simulink model "Sistema"  (R2023a)
settings: Solver=VariableStepAuto  StartTime=0.0  StopTime=15  MaxStep=1E-3  RelTol=1e-3
libraries: fl_lib x21, nesl_utility x9, slpidlib x2
settings Model: LastModifiedBy=vania
settings DataIOCC: SaveFormat=Array  ReturnWorkspaceOutputs=off  TimeSaveName=t
settings DebuggingCC: AlgebraicLoopMsg=none  ArtificialAlgebraicLoopMsg=none  MaxConsecutiveZCsMsg=none  ModelReferenceExtraNoncontSigs=none  OperatingPointInterfaceChecksumMismatchMsg=none
settings RTWCC: GPUComputeCapability=5.0

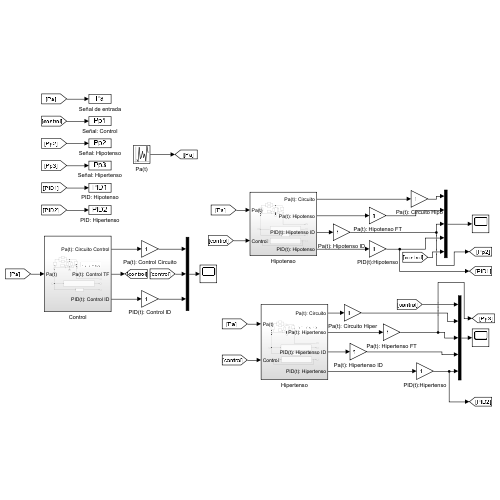
[thumbnail: Simulink's stored preview of the top-level diagram]
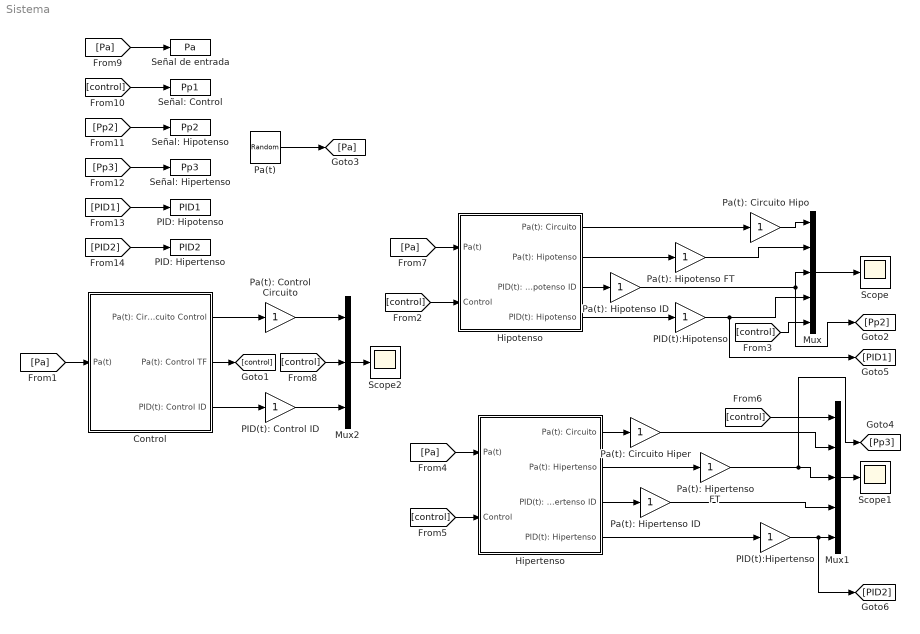
== system Sistema ==
  Control : Subsystem
  Hipertenso : Subsystem
  Hipotenso : Subsystem
  Mux : Mux  Inputs=5
  Mux1 : Mux  Inputs=5
  Mux2 : Mux  Inputs=3
  PID(t): Control ID : Gain
  PID(t):Hipertenso : Gain
  PID(t):Hipotenso : Gain
  PID: Hipertenso : ToWorkspace  VariableName=PID2  SampleTime=-1
  PID: Hipotenso : ToWorkspace  VariableName=PID1  SampleTime=-1
  Pa(t) : UniformRandomNumber  Minimum=-0.2  Seed=106  SampleTime=0.5
  Pa(t): Circuito Hiper : Gain
  Pa(t): Circuito Hipo : Gain
  Pa(t): Control Circuito : Gain
  Pa(t): Hipertenso FT : Gain
  Pa(t): Hipertenso ID : Gain
  Pa(t): Hipotenso FT : Gain
  Pa(t): Hipotenso ID : Gain
  Scope : Scope
  Scope1 : Scope
  Scope2 : Scope
  Señal de entrada : ToWorkspace  VariableName=Pa  SampleTime=-1
  Señal: Control : ToWorkspace  VariableName=Pp1  SampleTime=-1
  Señal: Hipertenso : ToWorkspace  VariableName=Pp3  SampleTime=-1
  Señal: Hipotenso : ToWorkspace  VariableName=Pp2  SampleTime=-1
  wires:
  Pa(t)/1 -> [Pa]
  Mux/1 -> Scope/1
  Hipotenso/1(Pa(t): Circuito) -> Pa(t): Circuito Hipo/1
  Hipotenso/2(Pa(t): Hipotenso) -> Pa(t): Hipotenso FT/1
  Hipotenso/3(PID(t): Hipotenso ID) -> Pa(t): Hipotenso ID/1
  Hipotenso/4(PID(t): Hipotenso) -> PID(t):Hipotenso/1
  [control] -> Hipotenso/2(Control)
  [control] -> Mux/5
  Pa(t): Hipotenso FT/1 -> Mux/2
  Pa(t): Circuito Hipo/1 -> Mux/1
  Pa(t): Hipotenso ID/1 -> Mux/3, [Pp2]
  PID(t):Hipotenso/1 -> Mux/4, [PID1]
  [Pa] -> Hipertenso/1(Pa(t))
  [control] -> Hipertenso/2(Control)
  Pa(t): Circuito Hiper/1 -> Mux1/2
  Hipertenso/1(Pa(t): Circuito) -> Pa(t): Circuito Hiper/1
  Hipertenso/2(Pa(t): Hipertenso) -> Pa(t): Hipertenso FT/1
  Pa(t): Hipertenso FT/1 -> [Pp3], Mux1/3
  Pa(t): Hipertenso ID/1 -> Mux1/4
  Hipertenso/3(PID(t): Hipertenso ID) -> Pa(t): Hipertenso ID/1
  PID(t):Hipertenso/1 -> [PID2], Mux1/5
  Hipertenso/4(PID(t): Hipertenso) -> PID(t):Hipertenso/1
  Mux1/1 -> Scope1/1
  [control] -> Mux1/1
  Mux2/1 -> Scope2/1
  [Pa] -> Control/1(Pa(t))
  [control] -> Mux2/2
  Control/2(Pa(t): Control TF) -> [control]
  [Pa] -> Hipotenso/1(Pa(t))
  PID(t): Control ID/1 -> Mux2/3
  Control/3(PID(t): Control ID) -> PID(t): Control ID/1
  Pa(t): Control Circuito/1 -> Mux2/1
  Control/1(Pa(t): Circuito Control) -> Pa(t): Control Circuito/1
  [Pa] -> Señal de entrada/1
  [control] -> Señal: Control/1
  [Pp2] -> Señal: Hipotenso/1
  [Pp3] -> Señal: Hipertenso/1
  [PID1] -> PID: Hipotenso/1
  [PID2] -> PID: Hipertenso/1

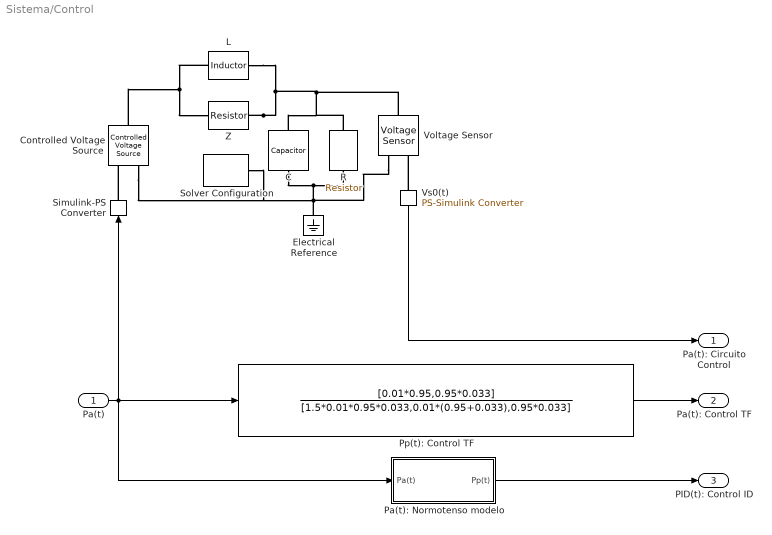
== system Sistema/Control ==
  Pa(t) : Inport
  C : fl_lib/Electrical/Electrical Elements/Capacitor  c=1.5 F  r=1e-6 Ohm  g=0 1/Ohm  i_specify=off  i_priority=None  i=0 A  i_nominal_specify=off  i_nominal_unit=A  i_nominal_value=1  v_specify=off  v_priority=None  v=0 V  v_nominal_specify=off  v_nominal_unit=V  v_nominal_value=1  vc_specify=off  vc_priority=High  vc=0 V  vc_nominal_specify=off  vc_nominal_unit=V  vc_nominal_value=1
  Controlled Voltage Source : fl_lib/Electrical/Electrical Sources/Controlled Voltage Source
  Electrical Reference : fl_lib/Electrical/Electrical Elements/Electrical Reference
  L : fl_lib/Electrical/Electrical Elements/Inductor  l=0.01 H  r=0 Ohm  g=1e-9 1/Ohm  i_specify=off  i_priority=None  i=0 A  i_nominal_specify=off  i_nominal_unit=A  i_nominal_value=1  v_specify=off  v_priority=None  v=0 V  v_nominal_specify=off  v_nominal_unit=V  v_nominal_value=1  i_L_specify=off  i_L_priority=High  i_L=0 A  i_L_nominal_specify=off  i_L_nominal_unit=A  i_L_nominal_value=1
  Pa(t): Normotenso modelo : Subsystem
  Pp(t): Control TF : TransferFcn  Numerator=[0.01*0.95,0.95*0.033]  Denominator=[1.5*0.01*0.95*0.033,0.01*(0.95+0.033),0.95*0.033]
  R : fl_lib/Electrical/Electrical Elements/Resistor  R=0.95 Ohm  i_specify=off  i_priority=None  i=0 A  i_nominal_specify=off  i_nominal_unit=A  i_nominal_value=1  v_specify=off  v_priority=None  v=0 V  v_nominal_specify=off  v_nominal_unit=V  v_nominal_value=1
  Simulink-PS Converter : nesl_utility/Simulink-PS Converter  PhysicalDomain=network_engine_domain  SubClassName=ps_input  LeftPortType=input  RightPortType=output  PseudoPeriodic=off  Frequencies=[]  NoiseDistribution=none  NoiseParameters=[]  Unit=1  AffineConversion=off  FilteringAndDerivatives=provide  SimscapeFilterOrder=1  InputFilterTimeConstant=0.001  UdotUserProvided=0
  Solver Configuration : nesl_utility/Solver Configuration  PhysicalDomain=network_engine_domain  SubClassName=solver  LeftPortType=input  RightPortType=generic  Tones=[]  Harmonics=[]  SimulateNoise=off  Profile=off  UseLocalSampling=off  EnableSwitchedLinearOptims=on  FrequencyDomain=off  UseCCode=off  RelTol=0.001  AbsTol=0.001  MinStep=1e-09  ToWorkspace=off  RevertToSquareIcSolve=off  NumHomotopyIterations=100  PhasorMode=off  PhasorModeNumHarmonics=1  ConsistencySolver=NEWTON_XTOL_AFTER_FTOL  IndexReductionMethod=DerivativeReplacement  DoDC=off  ResidualTolerance=1e-09  ConsistencyTolSource=GLOBAL  ConsistencyAbsTol=0.001  ConsistencyRelTol=0.001  ConsistencyTolFactor=0.001  UseLocalSolver=off  LocalSolverChoice=NE_BACKWARD_EULER_ADVANCER  ResolveIndetEquations=on  FunctionEvalNumThread=1  LocalSolverSampleTime=0.001  DoFixedCost=off  MaxNonlinIter=3  MaxModeIter=2  ComputeImpulses=off  ImpulseIterations=2  LinearAlgebra=auto  LinearAlgebraNumThread=0  EquationFormulation=NE_TIME_EF  DelaysMemoryBudget=1024  AutomaticFiltering=on  FilteringTimeConstant=0.001  PartitionStorageMethod=AS_NEEDED  PartitionMemoryBudget=1024  PartitionMethod=ROBUST
  Voltage Sensor : fl_lib/Electrical/Electrical Sensors/Voltage Sensor
  Vs0(t) : nesl_utility/PS-Simulink Converter  PhysicalDomain=network_engine_domain  SubClassName=ps_output  LeftPortType=input  RightPortType=output  PseudoPeriodic=off  Frequencies=[]  VectorFormat=1-D array  Unit=inherit  AffineConversion=off
  Z : fl_lib/Electrical/Electrical Elements/Resistor  R=0.033 Ohm  i_specify=off  i_priority=None  i=0 A  i_nominal_specify=off  i_nominal_unit=A  i_nominal_value=1  v_specify=off  v_priority=None  v=0 V  v_nominal_specify=off  v_nominal_unit=V  v_nominal_value=1
  Pa(t): Circuito Control : Outport
  Pa(t): Control TF : Outport  Port=2
  PID(t): Control ID : Outport  Port=3
  wires:
  Vs0(t)/1 -> Pa(t): Circuito Control/1
  Pp(t): Control TF/1 -> Pa(t): Control TF/1
  Pa(t)/1 -> Pp(t): Control TF/1, Pa(t): Normotenso modelo/1(Pa(t)), Simulink-PS Converter/1
  Pa(t): Normotenso modelo/1(Pp(t)) -> PID(t): Control ID/1
  connections:
  Vs0(t)/LConn1 -- Voltage Sensor/RConn1
  Simulink-PS Converter/RConn1 -- Controlled Voltage Source/RConn1
  L/LConn1 -- Controlled Voltage Source/LConn1 -- Z/LConn1
  Z/RConn1 -- L/RConn1 -- C/LConn1 -- R/LConn1 -- Voltage Sensor/LConn1
  Voltage Sensor/RConn2 -- Electrical Reference/LConn1 -- C/RConn1 -- R/RConn1 -- Solver Configuration/RConn1 -- Controlled Voltage Source/RConn2

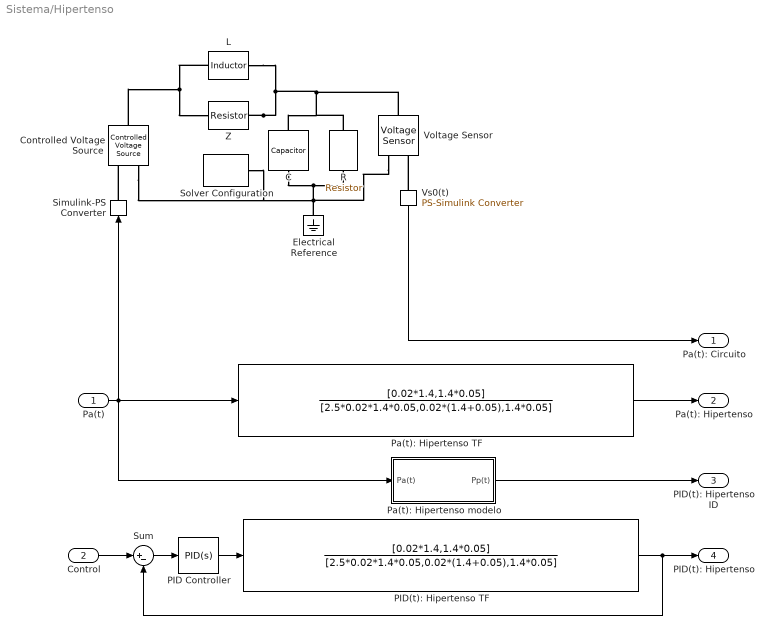
== system Sistema/Hipertenso ==
  Pa(t) : Inport
  Control : Inport  Port=2
  C : fl_lib/Electrical/Electrical Elements/Capacitor  c=2.5 F  r=1e-6 Ohm  g=0 1/Ohm  i_specify=off  i_priority=None  i=0 A  i_nominal_specify=off  i_nominal_unit=A  i_nominal_value=1  v_specify=off  v_priority=None  v=0 V  v_nominal_specify=off  v_nominal_unit=V  v_nominal_value=1  vc_specify=off  vc_priority=High  vc=0 V  vc_nominal_specify=off  vc_nominal_unit=V  vc_nominal_value=1
  Controlled Voltage Source : fl_lib/Electrical/Electrical Sources/Controlled Voltage Source
  Electrical Reference : fl_lib/Electrical/Electrical Elements/Electrical Reference
  L : fl_lib/Electrical/Electrical Elements/Inductor  l=0.02 H  r=0 Ohm  g=1e-9 1/Ohm  i_specify=off  i_priority=None  i=0 A  i_nominal_specify=off  i_nominal_unit=A  i_nominal_value=1  v_specify=off  v_priority=None  v=0 V  v_nominal_specify=off  v_nominal_unit=V  v_nominal_value=1  i_L_specify=off  i_L_priority=High  i_L=0 A  i_L_nominal_specify=off  i_L_nominal_unit=A  i_L_nominal_value=1
  PID Controller : slpidlib/PID Controller  Controller=PID  Form=Parallel  TimeDomain=Continuous-time  UseExternalTs=off  SampleTime=-1  IntegratorMethod=Forward Euler  FilterMethod=Forward Euler  ControllerParametersSource=internal  P=161.301085142962  I=38537.6348483401  UseKiTs=off  D=0.0221134918099117  N=4928.25992680153  UseFilter=on  TunerSelectOption=Transfer Function Based (PID Tuner App)  InitialConditionSource=internal  InitialConditionForIntegrator=0  InitialConditionForFilter=0  DifferentiatorICPrevScaledInput=0  ExternalReset=none  TrackingMode=off  Kt=1  LimitOutput=off  SatLimitsSource=internal  UpperSaturationLimit=inf  LowerSaturationLimit=-inf  LinearizeAsGain=on  AntiWindupMode=none  Kb=1  LimitIntegrator=off  UpperIntegratorSaturationLimit=inf  LowerIntegratorSaturationLimit=-inf  POutMin=[]  POutMax=[]  IOutMin=[]  IOutMax=[]  DOutMin=[]  DOutMax=[]  NOutMin=[]  NOutMax=[]  SumOutMin=[]  SumOutMax=[]  SaturationOutMin=[]  SaturationOutMax=[]  PParamMin=[]  PParamMax=[]  IParamMin=[]  IParamMax=[]  DParamMin=[]  DParamMax=[]  NParamMin=[]  NParamMax=[]  KbParamMin=[]  KbParamMax=[]  KtParamMin=[]  KtParamMax=[]  KbOutMin=[]  KbOutMax=[]  KtOutMin=[]  KtOutMax=[]  IntegratorOutMin=[]  IntegratorOutMax=[]  FilterOutMin=[]  FilterOutMax=[]  SumI1OutMin=[]  SumI1OutMax=[]  SumI2OutMin=[]  SumI2OutMax=[]  SumI3OutMin=[]  SumI3OutMax=[]  SumI4OutMin=[]  SumI4OutMax=[]  SumDOutMin=[]  SumDOutMax=[]  DifferentiatorOutMin=[]  DifferentiatorOutMax=[]  FilterDiffOutCoefMin=[]  FilterDiffOutCoefMax=[]  ReciprocalOutMin=[]  ReciprocalOutMax=[]  SumDenOutMin=[]  SumDenOutMax=[]  SumNumOutMin=[]  SumNumOutMax=[]  DivideOutMin=[]  DivideOutMax=[]  UdiffTsProdOutMin=[]  UdiffTsProdOutMax=[]  NTsProdOutMin=[]  NTsProdOutMax=[]  UintegralTsProdOutMin=[]  UintegralTsProdOutMax=[]  UngainTsProdOutMin=[]  UngainTsProdOutMax=[]  ClampingZeroOutDataTypeStr=Inherit: Inherit via back propagation  ClampingZeroOutMin=[]  ClampingZeroOutMax=[]  FilterDenConstantOutDataTypeStr=Inherit: Inherit via back propagation  FilterDenConstantOutMin=[]  FilterDenConstantOutMax=[]  PCopyOutDataTypeStr=Inherit: Inherit via back propagation  PCopyOutMin=[]  PCopyOutMax=[]  NCopyOutDataTypeStr=Inherit: Inherit via back propagation  NCopyOutMin=[]  NCopyOutMax=[]  IntegratorContinuousStateAttributes=''  IntegratorStateMustResolveToSignalObject=off  IntegratorRTWStateStorageClass=Auto  FilterContinuousStateAttributes=''  FilterStateMustResolveToSignalObject=off  FilterRTWStateStorageClass=Auto  ParallelPVariant=InternalParameters  IdealPVariant=Disabled  IVariant=InternalParameters  DVariant=InternalParameters  IntegratorVariant=Continuous  SatVariant=Disabled  AWVariant=Passthrough  PCopyVariant=Disabled  TRVariant=Disabled  FdbkBlocksVariant=Forward  IdealPFdbkVariant=Disabled  SatFdbkVariant=Disabled  DerivativeFilterVariant=ContFilter  NVariant=InternalParameters  NCopyVariant=Disabled  FilterICVariant=InternalICsFilter  IntegratorICVariant=InternalICs  ExternalResetVariant=Disabled  TRSumVariant=Passthrough  SumFdbkVariant=Disabled  SumVariant=Sum_PID  TsampFilterVariant=InternalTs  TsampNgainVariant=Passthrough  TsampIntegralVariant=Disabled_SignalSpec  ExternalSaturationOutDataTypeStr=Inherit: Same as second input
  PID(t): Hipertenso TF : TransferFcn  Numerator=[0.02*1.4,1.4*0.05]  Denominator=[2.5*0.02*1.4*0.05,0.02*(1.4+0.05),1.4*0.05]
  Pa(t): Hipertenso TF : TransferFcn  Numerator=[0.02*1.4,1.4*0.05]  Denominator=[2.5*0.02*1.4*0.05,0.02*(1.4+0.05),1.4*0.05]
  Pa(t): Hipertenso modelo : Subsystem
  R : fl_lib/Electrical/Electrical Elements/Resistor  R=1.4 Ohm  i_specify=off  i_priority=None  i=0 A  i_nominal_specify=off  i_nominal_unit=A  i_nominal_value=1  v_specify=off  v_priority=None  v=0 V  v_nominal_specify=off  v_nominal_unit=V  v_nominal_value=1
  Simulink-PS Converter : nesl_utility/Simulink-PS Converter  PhysicalDomain=network_engine_domain  SubClassName=ps_input  LeftPortType=input  RightPortType=output  PseudoPeriodic=off  Frequencies=[]  NoiseDistribution=none  NoiseParameters=[]  Unit=1  AffineConversion=off  FilteringAndDerivatives=provide  SimscapeFilterOrder=1  InputFilterTimeConstant=0.001  UdotUserProvided=0
  Solver Configuration : nesl_utility/Solver Configuration  PhysicalDomain=network_engine_domain  SubClassName=solver  LeftPortType=input  RightPortType=generic  Tones=[]  Harmonics=[]  SimulateNoise=off  Profile=off  UseLocalSampling=off  EnableSwitchedLinearOptims=on  FrequencyDomain=off  UseCCode=off  RelTol=0.001  AbsTol=0.001  MinStep=1e-09  ToWorkspace=off  RevertToSquareIcSolve=off  NumHomotopyIterations=100  PhasorMode=off  PhasorModeNumHarmonics=1  ConsistencySolver=NEWTON_XTOL_AFTER_FTOL  IndexReductionMethod=DerivativeReplacement  DoDC=off  ResidualTolerance=1e-09  ConsistencyTolSource=GLOBAL  ConsistencyAbsTol=0.001  ConsistencyRelTol=0.001  ConsistencyTolFactor=0.001  UseLocalSolver=off  LocalSolverChoice=NE_BACKWARD_EULER_ADVANCER  ResolveIndetEquations=on  FunctionEvalNumThread=1  LocalSolverSampleTime=0.001  DoFixedCost=off  MaxNonlinIter=3  MaxModeIter=2  ComputeImpulses=off  ImpulseIterations=2  LinearAlgebra=auto  LinearAlgebraNumThread=0  EquationFormulation=NE_TIME_EF  DelaysMemoryBudget=1024  AutomaticFiltering=on  FilteringTimeConstant=0.001  PartitionStorageMethod=AS_NEEDED  PartitionMemoryBudget=1024  PartitionMethod=ROBUST
  Sum : Sum  Inputs=|+-
  Voltage Sensor : fl_lib/Electrical/Electrical Sensors/Voltage Sensor
  Vs0(t) : nesl_utility/PS-Simulink Converter  PhysicalDomain=network_engine_domain  SubClassName=ps_output  LeftPortType=input  RightPortType=output  PseudoPeriodic=off  Frequencies=[]  VectorFormat=1-D array  Unit=inherit  AffineConversion=off
  Z : fl_lib/Electrical/Electrical Elements/Resistor  R=0.05 Ohm  i_specify=off  i_priority=None  i=0 A  i_nominal_specify=off  i_nominal_unit=A  i_nominal_value=1  v_specify=off  v_priority=None  v=0 V  v_nominal_specify=off  v_nominal_unit=V  v_nominal_value=1
  Pa(t): Circuito : Outport
  Pa(t): Hipertenso : Outport  Port=2
  PID(t): Hipertenso ID : Outport  Port=3
  PID(t): Hipertenso : Outport  Port=4
  wires:
  Sum/1 -> PID Controller/1
  PID Controller/1 -> PID(t): Hipertenso TF/1
  PID(t): Hipertenso TF/1 -> PID(t): Hipertenso/1, Sum/2
  Vs0(t)/1 -> Pa(t): Circuito/1
  Pa(t): Hipertenso TF/1 -> Pa(t): Hipertenso/1
  Pa(t)/1 -> Pa(t): Hipertenso TF/1, Pa(t): Hipertenso modelo/1(Pa(t)), Simulink-PS Converter/1
  Control/1 -> Sum/1
  Pa(t): Hipertenso modelo/1(Pp(t)) -> PID(t): Hipertenso ID/1
  connections:
  Vs0(t)/LConn1 -- Voltage Sensor/RConn1
  Simulink-PS Converter/RConn1 -- Controlled Voltage Source/RConn1
  L/LConn1 -- Controlled Voltage Source/LConn1 -- Z/LConn1
  Z/RConn1 -- L/RConn1 -- C/LConn1 -- R/LConn1 -- Voltage Sensor/LConn1
  Voltage Sensor/RConn2 -- Electrical Reference/LConn1 -- C/RConn1 -- R/RConn1 -- Solver Configuration/RConn1 -- Controlled Voltage Source/RConn2

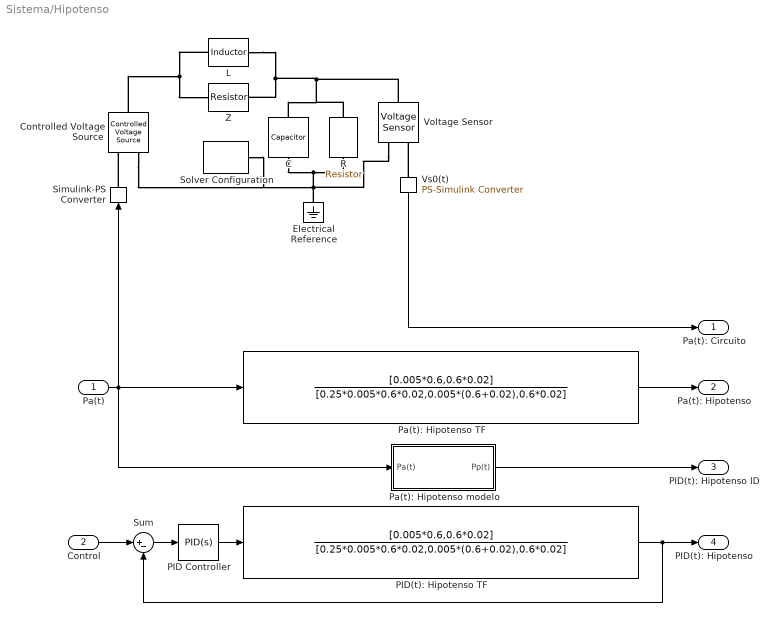
== system Sistema/Hipotenso ==
  Pa(t) : Inport
  Control : Inport  Port=2
  C : fl_lib/Electrical/Electrical Elements/Capacitor  c=0.25 F  r=1e-6 Ohm  g=0 1/Ohm  i_specify=off  i_priority=None  i=0 A  i_nominal_specify=off  i_nominal_unit=A  i_nominal_value=1  v_specify=off  v_priority=None  v=0 V  v_nominal_specify=off  v_nominal_unit=V  v_nominal_value=1  vc_specify=off  vc_priority=High  vc=0 V  vc_nominal_specify=off  vc_nominal_unit=V  vc_nominal_value=1
  Controlled Voltage Source : fl_lib/Electrical/Electrical Sources/Controlled Voltage Source
  Electrical Reference : fl_lib/Electrical/Electrical Elements/Electrical Reference
  L : fl_lib/Electrical/Electrical Elements/Inductor  l=0.005 H  r=0 Ohm  g=1e-9 1/Ohm  i_specify=off  i_priority=None  i=0 A  i_nominal_specify=off  i_nominal_unit=A  i_nominal_value=1  v_specify=off  v_priority=None  v=0 V  v_nominal_specify=off  v_nominal_unit=V  v_nominal_value=1  i_L_specify=off  i_L_priority=High  i_L=0 A  i_L_nominal_specify=off  i_L_nominal_unit=A  i_L_nominal_value=1
  PID Controller : slpidlib/PID Controller  Controller=PID  Form=Parallel  TimeDomain=Continuous-time  UseExternalTs=off  SampleTime=-1  IntegratorMethod=Forward Euler  FilterMethod=Forward Euler  ControllerParametersSource=internal  P=1.49397900518606  I=352.000659394334  UseKiTs=off  D=0.00049119206492278  N=536.918505743178  UseFilter=on  TunerSelectOption=Transfer Function Based (PID Tuner App)  InitialConditionSource=internal  InitialConditionForIntegrator=0  InitialConditionForFilter=0  DifferentiatorICPrevScaledInput=0  ExternalReset=none  TrackingMode=off  Kt=1  LimitOutput=off  SatLimitsSource=internal  UpperSaturationLimit=inf  LowerSaturationLimit=-inf  LinearizeAsGain=on  AntiWindupMode=none  Kb=1  LimitIntegrator=off  UpperIntegratorSaturationLimit=inf  LowerIntegratorSaturationLimit=-inf  POutMin=[]  POutMax=[]  IOutMin=[]  IOutMax=[]  DOutMin=[]  DOutMax=[]  NOutMin=[]  NOutMax=[]  SumOutMin=[]  SumOutMax=[]  SaturationOutMin=[]  SaturationOutMax=[]  PParamMin=[]  PParamMax=[]  IParamMin=[]  IParamMax=[]  DParamMin=[]  DParamMax=[]  NParamMin=[]  NParamMax=[]  KbParamMin=[]  KbParamMax=[]  KtParamMin=[]  KtParamMax=[]  KbOutMin=[]  KbOutMax=[]  KtOutMin=[]  KtOutMax=[]  IntegratorOutMin=[]  IntegratorOutMax=[]  FilterOutMin=[]  FilterOutMax=[]  SumI1OutMin=[]  SumI1OutMax=[]  SumI2OutMin=[]  SumI2OutMax=[]  SumI3OutMin=[]  SumI3OutMax=[]  SumI4OutMin=[]  SumI4OutMax=[]  SumDOutMin=[]  SumDOutMax=[]  DifferentiatorOutMin=[]  DifferentiatorOutMax=[]  FilterDiffOutCoefMin=[]  FilterDiffOutCoefMax=[]  ReciprocalOutMin=[]  ReciprocalOutMax=[]  SumDenOutMin=[]  SumDenOutMax=[]  SumNumOutMin=[]  SumNumOutMax=[]  DivideOutMin=[]  DivideOutMax=[]  UdiffTsProdOutMin=[]  UdiffTsProdOutMax=[]  NTsProdOutMin=[]  NTsProdOutMax=[]  UintegralTsProdOutMin=[]  UintegralTsProdOutMax=[]  UngainTsProdOutMin=[]  UngainTsProdOutMax=[]  ClampingZeroOutDataTypeStr=Inherit: Inherit via back propagation  ClampingZeroOutMin=[]  ClampingZeroOutMax=[]  FilterDenConstantOutDataTypeStr=Inherit: Inherit via back propagation  FilterDenConstantOutMin=[]  FilterDenConstantOutMax=[]  PCopyOutDataTypeStr=Inherit: Inherit via back propagation  PCopyOutMin=[]  PCopyOutMax=[]  NCopyOutDataTypeStr=Inherit: Inherit via back propagation  NCopyOutMin=[]  NCopyOutMax=[]  IntegratorContinuousStateAttributes=''  IntegratorStateMustResolveToSignalObject=off  IntegratorRTWStateStorageClass=Auto  FilterContinuousStateAttributes=''  FilterStateMustResolveToSignalObject=off  FilterRTWStateStorageClass=Auto  ParallelPVariant=InternalParameters  IdealPVariant=Disabled  IVariant=InternalParameters  DVariant=InternalParameters  IntegratorVariant=Continuous  SatVariant=Disabled  AWVariant=Passthrough  PCopyVariant=Disabled  TRVariant=Disabled  FdbkBlocksVariant=Forward  IdealPFdbkVariant=Disabled  SatFdbkVariant=Disabled  DerivativeFilterVariant=ContFilter  NVariant=InternalParameters  NCopyVariant=Disabled  FilterICVariant=InternalICsFilter  IntegratorICVariant=InternalICs  ExternalResetVariant=Disabled  TRSumVariant=Passthrough  SumFdbkVariant=Disabled  SumVariant=Sum_PID  TsampFilterVariant=InternalTs  TsampNgainVariant=Passthrough  TsampIntegralVariant=Disabled_SignalSpec  ExternalSaturationOutDataTypeStr=Inherit: Same as second input
  PID(t): Hipotenso TF : TransferFcn  Numerator=[0.005*0.6,0.6*0.02]  Denominator=[0.25*0.005*0.6*0.02,0.005*(0.6+0.02),0.6*0.02]
  Pa(t): Hipotenso TF : TransferFcn  Numerator=[0.005*0.6,0.6*0.02]  Denominator=[0.25*0.005*0.6*0.02,0.005*(0.6+0.02),0.6*0.02]
  Pa(t): Hipotenso modelo : Subsystem
  R : fl_lib/Electrical/Electrical Elements/Resistor  R=0.6 Ohm  i_specify=off  i_priority=None  i=0 A  i_nominal_specify=off  i_nominal_unit=A  i_nominal_value=1  v_specify=off  v_priority=None  v=0 V  v_nominal_specify=off  v_nominal_unit=V  v_nominal_value=1
  Simulink-PS Converter : nesl_utility/Simulink-PS Converter  PhysicalDomain=network_engine_domain  SubClassName=ps_input  LeftPortType=input  RightPortType=output  PseudoPeriodic=off  Frequencies=[]  NoiseDistribution=none  NoiseParameters=[]  Unit=1  AffineConversion=off  FilteringAndDerivatives=provide  SimscapeFilterOrder=1  InputFilterTimeConstant=0.001  UdotUserProvided=0
  Solver Configuration : nesl_utility/Solver Configuration  PhysicalDomain=network_engine_domain  SubClassName=solver  LeftPortType=input  RightPortType=generic  Tones=[]  Harmonics=[]  SimulateNoise=off  Profile=off  UseLocalSampling=off  EnableSwitchedLinearOptims=on  FrequencyDomain=off  UseCCode=off  RelTol=0.001  AbsTol=0.001  MinStep=1e-09  ToWorkspace=off  RevertToSquareIcSolve=off  NumHomotopyIterations=100  PhasorMode=off  PhasorModeNumHarmonics=1  ConsistencySolver=NEWTON_XTOL_AFTER_FTOL  IndexReductionMethod=DerivativeReplacement  DoDC=off  ResidualTolerance=1e-09  ConsistencyTolSource=GLOBAL  ConsistencyAbsTol=0.001  ConsistencyRelTol=0.001  ConsistencyTolFactor=0.001  UseLocalSolver=off  LocalSolverChoice=NE_BACKWARD_EULER_ADVANCER  ResolveIndetEquations=on  FunctionEvalNumThread=1  LocalSolverSampleTime=0.001  DoFixedCost=off  MaxNonlinIter=3  MaxModeIter=2  ComputeImpulses=off  ImpulseIterations=2  LinearAlgebra=auto  LinearAlgebraNumThread=0  EquationFormulation=NE_TIME_EF  DelaysMemoryBudget=1024  AutomaticFiltering=on  FilteringTimeConstant=0.001  PartitionStorageMethod=AS_NEEDED  PartitionMemoryBudget=1024  PartitionMethod=ROBUST
  Sum : Sum  Inputs=|+-
  Voltage Sensor : fl_lib/Electrical/Electrical Sensors/Voltage Sensor
  Vs0(t) : nesl_utility/PS-Simulink Converter  PhysicalDomain=network_engine_domain  SubClassName=ps_output  LeftPortType=input  RightPortType=output  PseudoPeriodic=off  Frequencies=[]  VectorFormat=1-D array  Unit=inherit  AffineConversion=off
  Z : fl_lib/Electrical/Electrical Elements/Resistor  R=0.02 Ohm  i_specify=off  i_priority=None  i=0 A  i_nominal_specify=off  i_nominal_unit=A  i_nominal_value=1  v_specify=off  v_priority=None  v=0 V  v_nominal_specify=off  v_nominal_unit=V  v_nominal_value=1
  Pa(t): Circuito : Outport
  Pa(t): Hipotenso : Outport  Port=2
  PID(t): Hipotenso ID : Outport  Port=3
  PID(t): Hipotenso : Outport  Port=4
  wires:
  Sum/1 -> PID Controller/1
  PID Controller/1 -> PID(t): Hipotenso TF/1
  PID(t): Hipotenso TF/1 -> PID(t): Hipotenso/1, Sum/2
  Vs0(t)/1 -> Pa(t): Circuito/1
  Pa(t): Hipotenso TF/1 -> Pa(t): Hipotenso/1
  Pa(t)/1 -> Pa(t): Hipotenso modelo/1(Pa(t)), Simulink-PS Converter/1, Pa(t): Hipotenso TF/1
  Control/1 -> Sum/1
  Pa(t): Hipotenso modelo/1(Pp(t)) -> PID(t): Hipotenso ID/1
  connections:
  Vs0(t)/LConn1 -- Voltage Sensor/RConn1
  Simulink-PS Converter/RConn1 -- Controlled Voltage Source/RConn1
  Controlled Voltage Source/LConn1 -- Z/LConn1 -- L/LConn1
  L/RConn1 -- Voltage Sensor/LConn1 -- C/LConn1 -- R/LConn1 -- Z/RConn1
  C/RConn1 -- Solver Configuration/RConn1 -- Controlled Voltage Source/RConn2 -- Voltage Sensor/RConn2 -- Electrical Reference/LConn1 -- R/RConn1

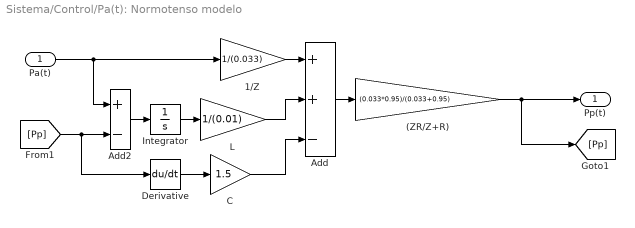
== system Sistema/Control/Pa(t): Normotenso modelo ==
  Pa(t) : Inport
  (ZR/Z+R) : Gain  Gain=(0.033*0.95)/(0.033+0.95)
  1/Z : Gain  Gain=1/(0.033)
  Add : Sum  Inputs=++-
  Add2 : Sum  Inputs=+-
  C : Gain  Gain=1.5
  Derivative : Derivative
  Integrator : Integrator
  L : Gain  Gain=1/(0.01)
  Pp(t) : Outport
  wires:
  1/Z/1 -> Add/1
  Pa(t)/1 -> Add2/1, 1/Z/1
  Integrator/1 -> L/1
  Add2/1 -> Integrator/1
  C/1 -> Add/3
  L/1 -> Add/2
  Derivative/1 -> C/1
  [Pp] -> Derivative/1, Add2/2
  Add/1 -> (ZR/Z+R)/1
  (ZR/Z+R)/1 -> [Pp], Pp(t)/1

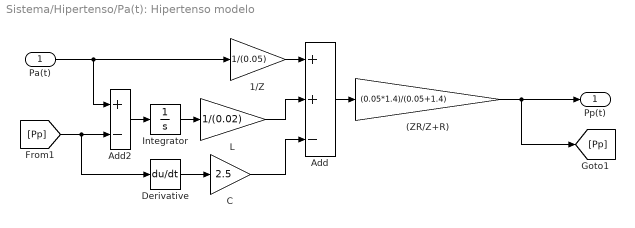
== system Sistema/Hipertenso/Pa(t): Hipertenso modelo ==
  Pa(t) : Inport
  (ZR/Z+R) : Gain  Gain=(0.05*1.4)/(0.05+1.4)
  1/Z : Gain  Gain=1/(0.05)
  Add : Sum  Inputs=++-
  Add2 : Sum  Inputs=+-
  C : Gain  Gain=2.5
  Derivative : Derivative
  Integrator : Integrator
  L : Gain  Gain=1/(0.02)
  Pp(t) : Outport
  wires:
  1/Z/1 -> Add/1
  Pa(t)/1 -> Add2/1, 1/Z/1
  Integrator/1 -> L/1
  Add2/1 -> Integrator/1
  C/1 -> Add/3
  L/1 -> Add/2
  Derivative/1 -> C/1
  [Pp] -> Derivative/1, Add2/2
  Add/1 -> (ZR/Z+R)/1
  (ZR/Z+R)/1 -> [Pp], Pp(t)/1

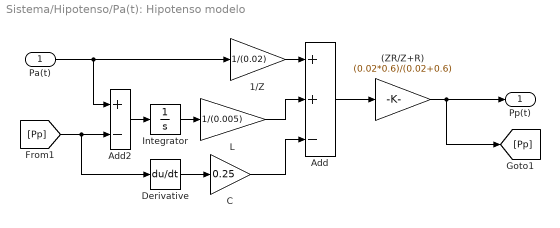
== system Sistema/Hipotenso/Pa(t): Hipotenso modelo ==
  Pa(t) : Inport
  (ZR/Z+R) : Gain  Gain=(0.02*0.6)/(0.02+0.6)
  1/Z : Gain  Gain=1/(0.02)
  Add : Sum  Inputs=++-
  Add2 : Sum  Inputs=+-
  C : Gain  Gain=0.25
  Derivative : Derivative
  Integrator : Integrator
  L : Gain  Gain=1/(0.005)
  Pp(t) : Outport
  wires:
  1/Z/1 -> Add/1
  Pa(t)/1 -> Add2/1, 1/Z/1
  Integrator/1 -> L/1
  Add2/1 -> Integrator/1
  C/1 -> Add/3
  L/1 -> Add/2
  Derivative/1 -> C/1
  [Pp] -> Derivative/1, Add2/2
  Add/1 -> (ZR/Z+R)/1
  (ZR/Z+R)/1 -> [Pp], Pp(t)/1
